simulink library "INT_StSys_TrqShutOff"  (R2016b)
settings: Solver=VariableStepAuto  StartTime=0.0  StopTime=10.0  RelTol=1e-3
settings Model: Creator=Administrator  LastModifiedBy=Administrator

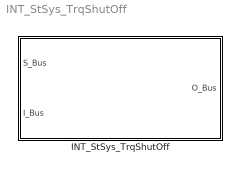
== system INT_StSys_TrqShutOff ==
  INT_StSys_TrqShutOff : Subsystem

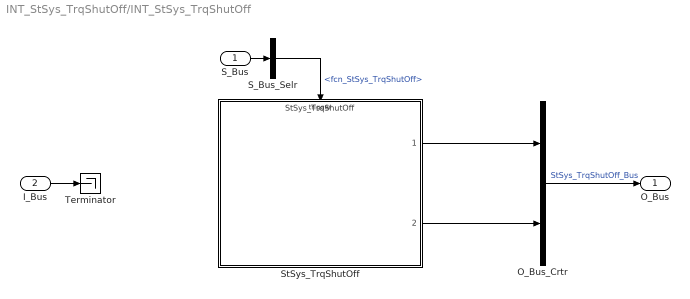
== system INT_StSys_TrqShutOff/INT_StSys_TrqShutOff ==
  S_Bus : Inport
  I_Bus : Inport  Port=2
  O_Bus_Crtr : BusCreator  Inputs=2
  S_Bus_Selr : BusSelector  OutputSignals=fcn_StSys_TrqShutOff
  StSys_TrqShutOff : ModelReference  ModelNameDialog=StSys_TrqShutOff  SimulationMode=Normal  ModelReferenceVersion=1.2  TriggerPortName=function  TriggerPortTriggerType=function-call  TriggerPortStatesWhenEnabling=held
  Terminator : Terminator
  O_Bus : Outport
  wires:
  S_Bus_Selr/1 -> StSys_TrqShutOff/Trigger  "<fcn_StSys_TrqShutOff>"
  S_Bus/1 -> S_Bus_Selr/1
  I_Bus/1 -> Terminator/1
  O_Bus_Crtr/1 -> O_Bus/1  "StSys_TrqShutOff_Bus"
  StSys_TrqShutOff/1 -> O_Bus_Crtr/1
  StSys_TrqShutOff/2 -> O_Bus_Crtr/2
